simulink model "Cruise_Control_dsgn"  (R2020b)
settings: Solver=VariableStepAuto  StartTime=0.0  StopTime=700  RelTol=1e-3
InitFcn:
  | Cruise_Control_design
values from neighbouring files (symbols this model uses):
  Kd = 1.2    [CACC_6_vehicles_with_independent_FF_of_LeadVeh_Acceltn_Pstn.m]    (also in CACC_init.m; Cruise_Control_design.m = 247.7833)
  Ki = 10.1187    [Cruise_Control_design.m]
  Kp = 1.5    [CACC_6_vehicles_with_independent_FF_of_LeadVeh_Acceltn_Pstn.m]    (also in CACC_init.m; Cruise_Control_design.m = 174.6119)
  m = 1084    [ACC_Script.m]    (also in Cruise_Control_design.m; Headway_Controller_Design.m; mpc_init.m = 1140)
  plant_num = 9.2251*1e-4    (= 0.00092251)    [ACC_Script.m]    (also in Cruise_Control_design.m; Headway_Controller_Design.m = 0.00092212)
  V_set_speed = str2double(answer)    [Cruise_Control_design.m]
libraries: pid_lib x1
settings Model: Creator=ChOm1  LastModifiedBy=ChOm1

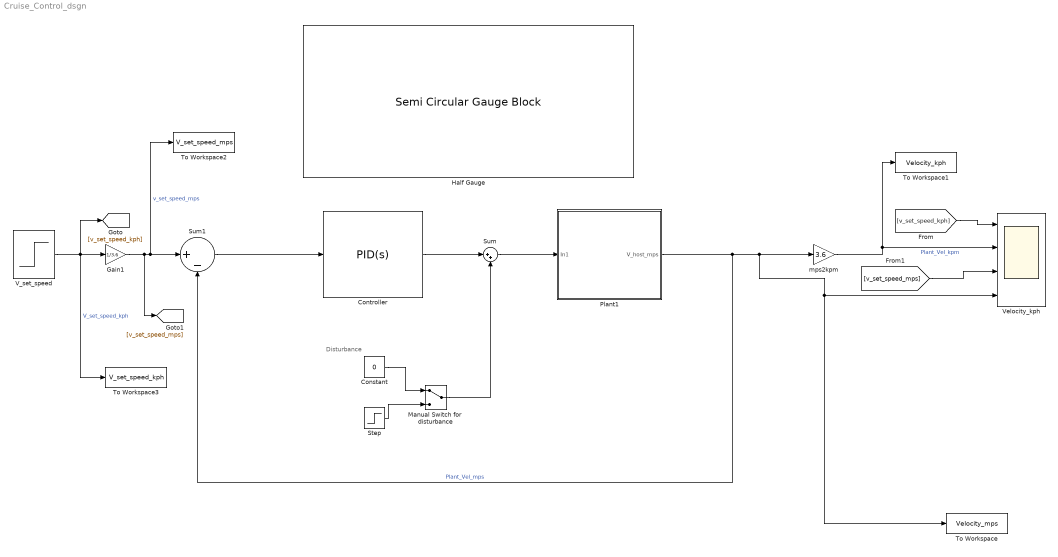
== system Cruise_Control_dsgn ==
  note: Disturbance
  Constant : Constant  Value=0
  Controller : pid_lib/PID Controller  Controller=PID  Form=Parallel  TimeDomain=Continuous-time  UseExternalTs=off  SampleTime=-1  IntegratorMethod=Forward Euler  FilterMethod=Forward Euler  ControllerParametersSource=internal  P=Kp  I=Ki  D=Kd  UseFilter=on  N=100  TunerSelectOption=Transfer Function Based (PID Tuner App)  InitialConditionSource=internal  InitialConditionForIntegrator=0  InitialConditionForFilter=0  DifferentiatorICPrevScaledInput=0  ExternalReset=none  TrackingMode=off  Kt=1  LimitOutput=off  SatLimitsSource=internal  UpperSaturationLimit=inf  LowerSaturationLimit=-inf  LinearizeAsGain=on  AntiWindupMode=none  Kb=1  POutMin=[]  POutMax=[]  IOutMin=[]  IOutMax=[]  DOutMin=[]  DOutMax=[]  NOutMin=[]  NOutMax=[]  SumOutMin=[]  SumOutMax=[]  SaturationOutMin=[]  SaturationOutMax=[]  PParamMin=[]  PParamMax=[]  IParamMin=[]  IParamMax=[]  DParamMin=[]  DParamMax=[]  NParamMin=[]  NParamMax=[]  KbParamMin=[]  KbParamMax=[]  KtParamMin=[]  KtParamMax=[]  KbOutMin=[]  KbOutMax=[]  KtOutMin=[]  KtOutMax=[]  IntegratorOutMin=[]  IntegratorOutMax=[]  FilterOutMin=[]  FilterOutMax=[]  SumI1OutMin=[]  SumI1OutMax=[]  SumI2OutMin=[]  SumI2OutMax=[]  SumI3OutMin=[]  SumI3OutMax=[]  SumI4OutMin=[]  SumI4OutMax=[]  SumDOutMin=[]  SumDOutMax=[]  DifferentiatorOutMin=[]  DifferentiatorOutMax=[]  FilterDiffOutCoefMin=[]  FilterDiffOutCoefMax=[]  ReciprocalOutMin=[]  ReciprocalOutMax=[]  SumDenOutMin=[]  SumDenOutMax=[]  SumNumOutMin=[]  SumNumOutMax=[]  DivideOutMin=[]  DivideOutMax=[]  UdiffTsProdOutMin=[]  UdiffTsProdOutMax=[]  NTsProdOutMin=[]  NTsProdOutMax=[]  UintegralTsProdOutMin=[]  UintegralTsProdOutMax=[]  UngainTsProdOutMin=[]  UngainTsProdOutMax=[]  IntegratorContinuousStateAttributes=''  IntegratorStateMustResolveToSignalObject=off  IntegratorRTWStateStorageClass=Auto  FilterContinuousStateAttributes=''  FilterStateMustResolveToSignalObject=off  FilterRTWStateStorageClass=Auto  ParallelPVariant=InternalParameters  IdealPVariant=Disabled  IVariant=InternalParameters  DVariant=InternalParameters  IntegratorVariant=Continuous  SatVariant=Disabled  AWVariant=Passthrough  PCopyVariant=Disabled  TRVariant=Disabled  FdbkBlocksVariant=Forward  IdealPFdbkVariant=Disabled  SatFdbkVariant=Disabled  DerivativeFilterVariant=ContFilter  NVariant=InternalParameters  NCopyVariant=Disabled  FilterICVariant=InternalICsFilter  IntegratorICVariant=InternalICs  ExternalResetVariant=Disabled  TRSumVariant=Passthrough  SumFdbkVariant=Disabled  SumVariant=Sum_PID  TsampFilterVariant=InternalTs  TsampNgainVariant=Passthrough  TsampIntegralVariant=Passthrough  ExternalSaturationOutDataTypeStr=Inherit: Same as second input
  Gain1 : Gain  Gain=1/3.6
  Half Gauge : SemiCircularGaugeBlock  ScaleMax=250
  Manual Switch for  disturbance : ManualSwitch
  Plant1 : Subsystem
  Step : Step  Time=100  After=m*9.81*sin(pi/45)  SampleTime=0
  Sum : Sum  Inputs=|++
  Sum1 : Sum  Inputs=|+-
  To Workspace : ToWorkspace  VariableName=Velocity_mps  SaveFormat=Timeseries  SampleTime=-1
  To Workspace1 : ToWorkspace  VariableName=Velocity_kph  SaveFormat=Timeseries  SampleTime=-1
  To Workspace2 : ToWorkspace  VariableName=V_set_speed_mps  SaveFormat=Timeseries  SampleTime=-1
  To Workspace3 : ToWorkspace  VariableName=V_set_speed_kph  SaveFormat=Timeseries  SampleTime=-1
  V_set_speed : Step  After=V_set_speed  SampleTime=0
  Velocity_kph : Scope  NumInputPorts=4
  mps2kpm : Gain  Gain=3.6
  wires:
  mps2kpm/1 -> To Workspace1/1, Velocity_kph/2  "Plant_Vel_kpm"
  Plant1/1(V_host_mps) -> Sum1/2, To Workspace/1, Velocity_kph/4, mps2kpm/1  "Plant_Vel_mps"
  Controller/1 -> Sum/1
  Sum/1 -> Plant1/1(In1)
  Constant/1 -> Manual Switch for  disturbance/1
  Step/1 -> Manual Switch for  disturbance/2
  Manual Switch for  disturbance/1 -> Sum/2
  Sum1/1 -> Controller/1
  V_set_speed/1 -> To Workspace3/1, [v_set_speed_kph], Gain1/1  "V_set_speed_kph"
  Gain1/1 -> Sum1/1, To Workspace2/1, [v_set_speed_mps]  "v_set_speed_mps"
  [v_set_speed_kph] -> Velocity_kph/1
  [v_set_speed_mps] -> Velocity_kph/3

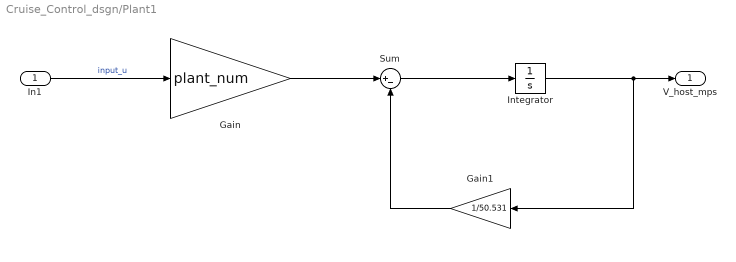
== system Cruise_Control_dsgn/Plant1 ==
  In1 : Inport
  Gain : Gain  Gain=plant_num
  Gain1 : Gain  Gain=1/50.531
  Integrator : Integrator
  Sum : Sum  Inputs=|+-
  V_host_mps : Outport
  wires:
  In1/1 -> Gain/1  "input_u"
  Gain/1 -> Sum/1
  Sum/1 -> Integrator/1
  Integrator/1 -> Gain1/1, V_host_mps/1
  Gain1/1 -> Sum/2
